simulink model "controlModel"  (R2024b)
settings: Solver=FixedStepAuto  StartTime=0.0  StopTime=inf  FixedStep=1e-3  RelTol=1e-3
values from neighbouring files (symbols this model uses):
  g = 9.806    [params.sldd]
  iamax = 10.0    [params.sldd]
  Kgain = 1.0    [params.sldd]
  phi0 = 0.1    [params.sldd]
  phisat = 0.5    [params.sldd]
  Ts = 0.001    [params.sldd]
  V0 = 0.1    [params.sldd]
  vmin = 1.0    [params.sldd]
undefined symbols (not defined in the file or in its folder): Discrete, Time
libraries: ctrlSharedLib x3, simulink x1
settings Model: DataDictionary=params.sldd  Creator=stefa  LastModifiedBy=lovaste79668
settings OptimizationCC: DefaultParameterBehavior=Inlined  UseDivisionForNetSlopeComputation=on  GainParamInheritBuiltInType=on  UseFloatMulNetSlope=on  UseSpecifiedMinMax=on  ReuseModelBlockBuffer=off  BitwiseOrLogicalOp=Bitwise operator  PassReuseOutputArgsAs=Individual arguments  ZeroExternalMemoryAtStartup=off  ZeroInternalMemoryAtStartup=off  NoFixptDivByZeroProtection=on  EfficientFloat2IntCast=on  LifeSpan=1  OptimizeBlockOrder=speed  DifferentSizesBufferReuse=on  EfficientTunableParamExpr=on
settings DebuggingCC: SignalInfNanChecking=warning  IntegerOverflowMsg=error  ParameterPrecisionLossMsg=none  ParameterTunabilityLossMsg=none  UnconnectedInputMsg=warning  UnconnectedOutputMsg=warning  UnconnectedLineMsg=warning  AssertControl=DisableAll  SFUndirectedBroadcastEventsDiag=error
settings HardwareCC: ProdBitPerPointer=32  ProdBitPerSizeT=32  ProdBitPerPtrDiffT=32  ProdLargestAtomicInteger=Long  ProdLargestAtomicFloat=Double  ProdWordSize=32  ProdLongLongMode=on  ProdHWDeviceType=ARM Compatible->ARM Cortex-M
settings ModelReferenceCC: EnableRefExpFcnMdlSchedulingChecks=on
settings SFSimCC: CompileTimeRecursionLimit=0  EnableRuntimeRecursion=off  MATLABDynamicMemAlloc=off  CustomCodeUndefinedFunction=UseInterfaceOnly  SimTargetLang=C++
settings RTWCC: Description=Embedded Coder  SystemTargetFile=ert.tlc  GenCodeOnly=on  TemplateMakefile=ert_default_tmf  GenerateReport=on  RTWUseSimCustomCode=on  Toolchain=CMake  LaunchReport=on  TargetLang=C++  GPUComputeCapability=3.5  DLArmComputeVersion=19.05
settings CodeAppCC: ForceParamTrailComments=on  IgnoreCustomStorageClasses=off  OperatorAnnotations=on  SimulinkDataObjDesc=on  SFDataObjDesc=on  MATLABFcnDesc=on  InsertBlockDesc=on
settings ERTTargetCC: TargetLangStandard=C++03 (ISO)  GenerateSampleERTMain=on  CombineSignalStateStructs=on  SuppressErrorStatus=on  CodeInterfacePackaging=C++ class  SupportComplex=off  ParenthesesLevel=Maximum  CastingMode=Standards  GenerateSharedConstants=off  InlinedParameterPlacement=Hierarchical  RootIOFormat=Structure reference  ERTCustomFileTemplate=example_file_process.tlc  EnableSignedLeftShifts=off  EnableSignedRightShifts=off  DynamicArrayContainerType=coder::array

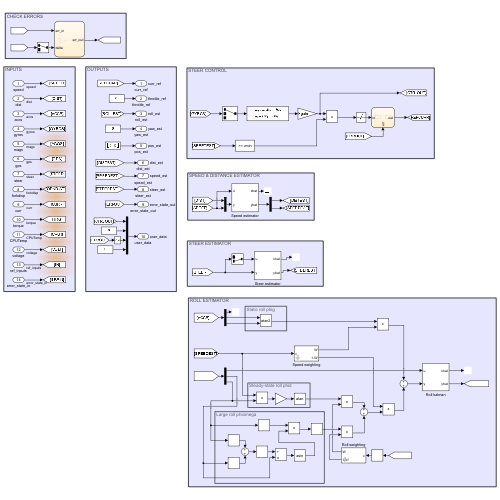
[thumbnail: Simulink's stored preview of the top-level diagram]
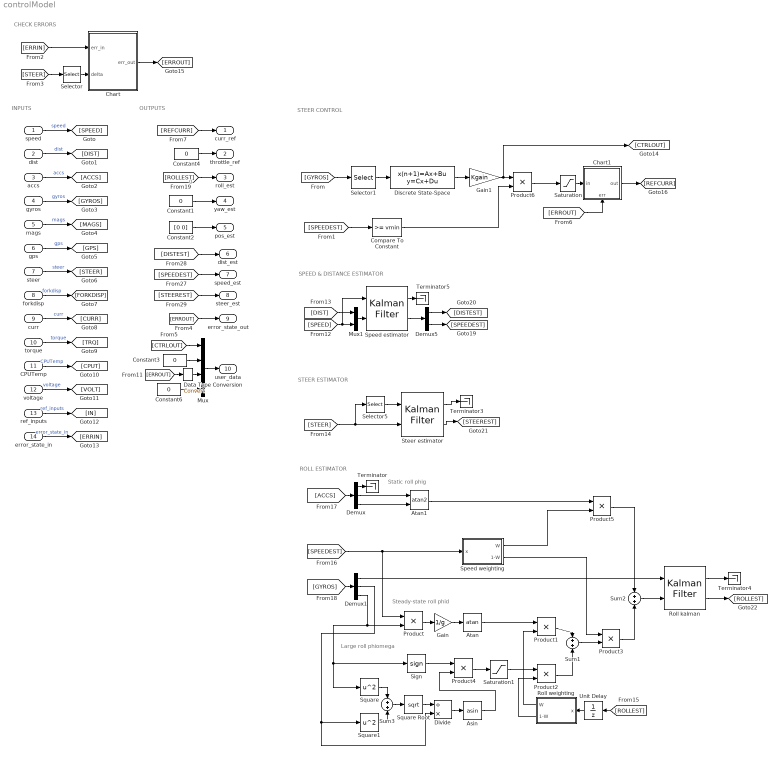
== system controlModel ==
  note: STEER CONTROL
  note: CHECK ERRORS
  note: OUTPUTS
  note: 0
  note: INPUTS
  note: SPEED & DISTANCE ESTIMATOR
  note: STEER ESTIMATOR
  note: Steady-state roll phid
  note: ROLL ESTIMATOR
  note: Static roll phig
  note: Large roll phiomega
  speed : Inport  OutDataTypeStr=single  PortDimensions=[1 1]
  dist : Inport  Port=2  OutDataTypeStr=single  PortDimensions=[1 1]
  accs : Inport  Port=3  OutDataTypeStr=single  PortDimensions=[3 1]
  gyros : Inport  Port=4  OutDataTypeStr=single  PortDimensions=[3 1]
  mags : Inport  Port=5  OutDataTypeStr=single  PortDimensions=[3 1]
  gps : Inport  Port=6  OutDataTypeStr=single  PortDimensions=[3 1]
  steer : Inport  Port=7  OutDataTypeStr=single  PortDimensions=[2 1]
  forkdisp : Inport  Port=8  OutDataTypeStr=single  PortDimensions=[1 1]
  curr : Inport  Port=9  OutDataTypeStr=single  PortDimensions=[1 1]
  torque : Inport  Port=10  OutDataTypeStr=single  PortDimensions=[1 1]
  CPUTemp : Inport  Port=11  OutDataTypeStr=single  PortDimensions=[1 1]
  voltage : Inport  Port=12  OutDataTypeStr=single  PortDimensions=[1 1]
  ref_inputs : Inport  Port=13  OutDataTypeStr=single  PortDimensions=[2 1]
  error_state_in : Inport  Port=14  OutDataTypeStr=uint8  PortDimensions=[1 1]
  Asin : Trigonometry  Operator=asin
  Atan : Trigonometry  Operator=atan
  Atan1 : Trigonometry  Operator=atan2
  Chart : Stateflow chart  TreatAsAtomicUnit=on
  Chart1 : Stateflow chart  TreatAsAtomicUnit=on
      settings: PortSchema="{\"entries\":[{\"content\":{\"sides\":[{\"content\":{\"connectorIds\":[\"In2\"]},\"type\":\"ConnectorPlacement.EquallySpacedRectSide\",\"uuid\":\"a7f247f2-f31a-4b26-82bd-1fe59a6d26c2\"},{\"content\":{\"connectorIds\":[\"Out1\"],\"side\":\"RIGHT\"},\"type\":\"ConnectorPlacement.EquallySpacedRectSide\",\"uuid\":\"fc5cfdaa-86ff-4983-b913-23b97ab75182\"},{\"content\":{\"connectorIds\":[],\"side\":\"TOP\"},\"type\":\"ConnectorPlacement.EquallySpacedRectSide\",\"uuid\":\"2e1bd19e-64ce-4ab8-b315-1349ef827ebc\"},{\"content\":{\"connectorIds\":[\"In1\"],\"side\":\"BOTTOM\"},\"type\":\"ConnectorPlacement.EquallySpacedRectSide\",\"uuid\":\"0b4ba65c-a8aa-4480-a2c1-0947fecb7059\"}]},\"type\":\"ConnectorPlacement.EquallySpacedConnector\",\"uuid\":\"dfa84f79-29f4-4b5c-9657-78f9d81deda5\"}],\"packageUris\":[\"http://schema.mathworks.com/mf0/Connector/R2020b\"],\"version\":\"1.0\"}"
  Compare To Constant : simulink/Logic and Bit Operations/Compare To Constant  relop=>=  const=vmin  OutDataTypeStr=boolean
  Constant{1,3..4,6} (4 alike) : Constant  Value=0  OutDataTypeStr=Inherit: Inherit via back propagation  SampleTime=-1
  Constant2 : Constant  Value=[0 0]  OutDataTypeStr=Inherit: Inherit via back propagation  SampleTime=-1
  Data Type Conversion : DataTypeConversion  SaturateOnIntegerOverflow=off  RndMeth=Floor
  Demux : Demux  Outputs=3
  Demux1 : Demux  Outputs=3
  Demux5 : Demux  Outputs=2
  Discrete State-Space : DiscreteStateSpace  A=Ksys{kctrl}.A  B=Ksys{kctrl}.B  C=Ksys{kctrl}.C  D=Ksys{kctrl}.D  SampleTime=-1
  Divide : Product  Inputs=/*
  Gain : Gain  Gain=1/g
  Gain1 : Gain  Gain=Kgain
  Mux : Mux
  Mux1 : Mux  Inputs=2
  Product{,1..6} (7 alike) : Product
  Roll kalman : ctrlSharedLib/Kalman Filter  TimeDomain=Discrete-Time  UseCurrentEstimator=on  ModelSource=Individual A, B, C, D matrices  ModelSourceVariable=ss(0.95,1,1,0,1)  A=[1, -Ts; 0, 1]  B=[Ts; 0]  C=[1, 0]  D=0  NumberOfStates=1  NumberOfInputs=1  NumberOfOutputs=1  InitialEstimateSource=Dialog  X0=0  P0=10  UseK=off  UseGH=off  NumberOfProcessNoiseInputs=1  G=1  TimeInvariantG=on  H=0  TimeInvariantH=on  Q=diag([5e-7, 1e-8])  TimeInvariantQ=on  R=0.5  TimeInvariantR=on  N=0  TimeInvariantN=on  AddInputPort=on  AddEnablePort=off  OutputEstimatedY=on  OutputP=off  Ts=-1
  Roll weighting : Subsystem  mask{x0=phi0}
      mask prompts: x0 "Reference value (x0)"
      mask DialogControl DescGroupVar Prompt: Exponential weight
      mask DialogControl DescTextVar Prompt: Exponential weight function with equation y=exp(-x^2/x0^2)
  Saturation : Saturate  UpperLimit=iamax  LowerLimit=-iamax
  Saturation1 : Saturate  UpperLimit=phisat  LowerLimit=-phisat
  Selector : Selector  IndexMode=Zero-based  InputPortWidth=2  IndexOptions=Index vector (dialog)  Indices=0  OutputSizes=1
  Selector1 : Selector  InputPortWidth=3  IndexOptions=Index vector (dialog)  Indices=1  OutputSizes=1
  Selector5 : Selector  IndexMode=Zero-based  InputPortWidth=2  IndexOptions=Index vector (dialog)  Indices=1  OutputSizes=1
  Sign : Signum
  Speed estimator : ctrlSharedLib/Kalman Filter  TimeDomain=Discrete-Time  UseCurrentEstimator=on  ModelSource=Individual A, B, C, D matrices  ModelSourceVariable=ss(0.95,1,1,0,1)  A=[1 Ts -Ts; 0 1 0; 0 0 1]  B=[0; 0; 0]  C=[1 0 0; 0 1 0]  D=[0; 0]  NumberOfStates=1  NumberOfInputs=1  NumberOfOutputs=1  InitialEstimateSource=Dialog  X0=0  P0=10  UseK=off  UseGH=off  NumberOfProcessNoiseInputs=1  G=1  TimeInvariantG=on  H=0  TimeInvariantH=on  Q=diag([1e-5 1e-5 1e-7])  TimeInvariantQ=on  R=diag([1e-4, 5e-2])  TimeInvariantR=on  N=0  TimeInvariantN=on  AddInputPort=on  AddEnablePort=off  OutputEstimatedY=on  OutputP=off  Ts=-1
  Speed weighting : Subsystem  mask{x0=V0}
      mask prompts: x0 "Reference value (x0)"
      mask DialogControl DescGroupVar Prompt: Exponential weight
      mask DialogControl DescTextVar Prompt: Exponential weight function with equation y=exp(-x^2/x0^2)
  Square : Math  Operator=square
  Square Root : Sqrt
  Square1 : Math  Operator=square
  Steer estimator : ctrlSharedLib/Kalman Filter  TimeDomain=Discrete-Time  UseCurrentEstimator=on  ModelSource=Individual A, B, C, D matrices  ModelSourceVariable=ss(0.95,1,1,0,1)  A=[1 Ts -Ts; 0 1 0; 0 0 1]  B=[0; 0; 0]  C=[1 0 0; 0 1 0]  D=[0; 0]  NumberOfStates=1  NumberOfInputs=1  NumberOfOutputs=1  InitialEstimateSource=Dialog  X0=0  P0=10  UseK=off  UseGH=off  NumberOfProcessNoiseInputs=1  G=1  TimeInvariantG=on  H=0  TimeInvariantH=on  Q=diag([1e-5 1e-5 1e-7])  TimeInvariantQ=on  R=diag([1e-3, 1e-2])  TimeInvariantR=on  N=0  TimeInvariantN=on  AddInputPort=on  AddEnablePort=off  OutputEstimatedY=on  OutputP=off  Ts=-1
  Sum1 : Sum  Inputs=+|+
  Sum2 : Sum  Inputs=+|+
  Sum3 : Sum  Inputs=+|+
  Terminator{,3..5} (4 alike) : Terminator
  Unit Delay : UnitDelay  SampleTime=-1  HasFrameUpgradeWarning=on
  curr_ref : Outport  SignalName=curr_ref  OutDataTypeStr=single  PortDimensions=[1 1]
  throttle_ref : Outport  Port=2  SignalName=throttle_ref  OutDataTypeStr=single  PortDimensions=[1 1]
  roll_est : Outport  Port=3  SignalName=roll_est  OutDataTypeStr=single  PortDimensions=[1 1]
  yaw_est : Outport  Port=4  SignalName=yaw_est  OutDataTypeStr=single  PortDimensions=[1 1]
  pos_est : Outport  Port=5  SignalName=pos_est  OutDataTypeStr=single  PortDimensions=[2 1]
  dist_est : Outport  Port=6  SignalName=dist_est  OutDataTypeStr=single  PortDimensions=[1 1]
  speed_est : Outport  Port=7  SignalName=speed_est  OutDataTypeStr=single  PortDimensions=[1 1]
  steer_est : Outport  Port=8  SignalName=steer_est  OutDataTypeStr=single  PortDimensions=[2 1]
  error_state_out : Outport  Port=9  SignalName=error_state_out  OutDataTypeStr=uint8  PortDimensions=[1 1]
  user_data : Outport  Port=10  SignalName=user_data  OutDataTypeStr=single  PortDimensions=[4 1]
  wires:
  Constant2/1 -> pos_est/1
  speed/1 -> [SPEED]  "speed"
  dist/1 -> [DIST]  "dist"
  accs/1 -> [ACCS]  "accs"
  gyros/1 -> [GYROS]  "gyros"
  mags/1 -> [MAGS]  "mags"
  gps/1 -> [GPS]  "gps"
  steer/1 -> [STEER]  "steer"
  forkdisp/1 -> [FORKDISP]  "forkdisp"
  curr/1 -> [CURR]  "curr"
  torque/1 -> [TRQ]  "torque"
  CPUTemp/1 -> [CPUT]  "CPUTemp"
  voltage/1 -> [VOLT]  "voltage"
  ref_inputs/1 -> [IN]  "ref_inputs"
  error_state_in/1 -> [ERRIN]  "error_state_in"
  Constant1/1 -> yaw_est/1
  [ROLLEST] -> roll_est/1
  Constant4/1 -> throttle_ref/1
  [REFCURR] -> curr_ref/1
  Mux/1 -> user_data/1
  Constant6/1 -> Mux/4
  [ERRIN] -> Chart/1(err_in)
  Chart/1(err_out) -> [ERROUT]
  [STEER] -> Selector/1
  Selector/1 -> Chart/2(delta)
  [ERROUT] -> error_state_out/1
  Saturation/1 -> Chart1/2(in)
  Chart1/1(out) -> [REFCURR]
  [ERROUT] -> Chart1/1(err)
  [CTRLOUT] -> Mux/1
  Constant3/1 -> Mux/2
  [ERROUT] -> Data Type Conversion/1
  Data Type Conversion/1 -> Mux/3
  Mux1/1 -> Speed estimator/2
  [DIST] -> Mux1/1
  Demux5/2 -> [SPEEDEST]
  [SPEED] -> Speed estimator/1, Mux1/2
  Demux5/1 -> [DISTEST]
  [STEER] -> Selector5/1, Steer estimator/2
  Selector5/1 -> Steer estimator/1
  Speed weighting/2(1-W) -> Product3/1
  [ROLLEST] -> Unit Delay/1
  Demux1/3 -> Product/2, Sign/1, Square/1
  Product3/1 -> Sum2/2
  Product1/1 -> Sum1/1
  Unit Delay/1 -> Roll weighting/1(x)
  Demux/3 -> Atan1/2
  Saturation1/1 -> Product2/1
  Asin/1 -> Product4/2
  Roll kalman/2 -> [ROLLEST]
  Product2/1 -> Sum1/2
  Atan1/1 -> Product5/1
  Sign/1 -> Product4/1
  Demux/2 -> Atan1/1
  Roll weighting/1(W) -> Product1/2
  Sum1/1 -> Product3/2
  Square/1 -> Sum3/1
  Square1/1 -> Sum3/2
  Demux1/2 -> Divide/2, Square1/1
  Roll weighting/2(1-W) -> Product2/2
  Demux1/1 -> Roll kalman/1
  Square Root/1 -> Divide/1
  Product4/1 -> Saturation1/1
  [SPEEDEST] -> Speed weighting/1(x), Product/1
  Atan/1 -> Product1/1
  Divide/1 -> Asin/1
  Product5/1 -> Sum2/1
  Sum2/1 -> Roll kalman/2
  Speed weighting/1(W) -> Product5/2
  Product/1 -> Gain/1
  Gain/1 -> Atan/1
  Sum3/1 -> Square Root/1
  [ACCS] -> Demux/1
  Demux/1 -> Terminator/1
  [GYROS] -> Demux1/1
  [DISTEST] -> dist_est/1
  [SPEEDEST] -> speed_est/1
  [STEEREST] -> steer_est/1
  Steer estimator/2 -> [STEEREST]
  Steer estimator/1 -> Terminator3/1
  Roll kalman/1 -> Terminator4/1
  Speed estimator/2 -> Demux5/1
  Speed estimator/1 -> Terminator5/1
  [SPEEDEST] -> Compare To Constant/1
  Compare To Constant/1 -> Product6/2
  Discrete State-Space/1 -> Gain1/1
  [GYROS] -> Selector1/1
  Selector1/1 -> Discrete State-Space/1
  Product6/1 -> Saturation/1
  Gain1/1 -> [CTRLOUT], Product6/1

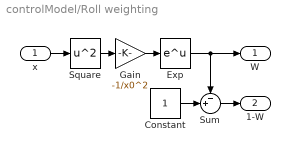
== system controlModel/Roll weighting ==
  x : Inport
  Constant : Constant  OutDataTypeStr=Inherit: Inherit via back propagation
  Exp : Math
  Gain : Gain  Gain=-1/x0^2
  Square : Math  Operator=square
  Sum : Sum  Inputs=-+|
  W : Outport
  1-W : Outport  Port=2
  wires:
  Gain/1 -> Exp/1
  Exp/1 -> Sum/1, W/1
  x/1 -> Square/1
  Square/1 -> Gain/1
  Constant/1 -> Sum/2
  Sum/1 -> 1-W/1

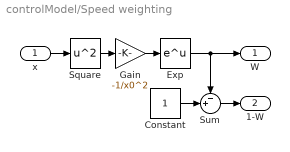
== system controlModel/Speed weighting ==
  x : Inport
  Constant : Constant  OutDataTypeStr=Inherit: Inherit via back propagation
  Exp : Math
  Gain : Gain  Gain=-1/x0^2
  Square : Math  Operator=square
  Sum : Sum  Inputs=-+|
  W : Outport
  1-W : Outport  Port=2
  wires:
  Gain/1 -> Exp/1
  Exp/1 -> Sum/1, W/1
  x/1 -> Square/1
  Square/1 -> Gain/1
  Constant/1 -> Sum/2
  Sum/1 -> 1-W/1

== stateflow chart controlModel/Chart1 ==
  state SETCURR
    out=in;
  state IDLE
    out=0;
  (default) -> SETCURR
  SETCURR -> SETCURR [order 2] : [err==0]
  SETCURR -> IDLE [order 1] : [err>0]
  IDLE -> IDLE
  data: err input uint8; in input single; out output single =single(0)

== stateflow chart controlModel/Chart ==
  state UPDATEERR
    err_out=err_in;
  state CHECKSTEER
    err_out=1;
  (default) -> UPDATEERR
  CHECKSTEER -> CHECKSTEER
  UPDATEERR -> (junction 32) : [err_out==0]
  (junction 32) -> CHECKSTEER [order 1] : [(abs(delta)>maxdelta)]
  (junction 32) -> UPDATEERR [order 2]
  data: err_in input uint8; delta input single; err_out output uint8; maxdelta parameter
